simulink model "Amp_baseline1"  (R2020a)
settings: Solver=ode45  StartTime=0.0  StopTime=60  RelTol=1e-3
model workspace (MAT data in the model file):
  cfg_native : object (value not decoded)
  en_add_channels = 1
  host_ip = 2130706433
  host_port = 50223
  local_ip = 2130706433
  local_port = 50224
  num_en_channels = 32
  num_samples = 1
  sample_rate = 250
  serial_number = 'NB-2015.10.93'
undefined symbols (not defined in the file or in its folder): A1, A138674, A30722, currentCFG_Amp_baseline_UB, D1, fdesignblkfcn, gcbh, I1, J138674, N30722, UB
libraries: gtecHighspeedLib x14, dspfdesign x3, dsparch4 x2, dspstat3 x1, TobiiEyeTrackerLib x1, gUSBamplib x1
settings Model: ModifiedByFormat=g.tec  Creator=g.tec medical engineering  LastModifiedBy=g.tec
settings DataIOCC: LimitDataPoints=on  SaveFormat=Array  ReturnWorkspaceOutputs=off
settings OptimizationCC: BlockReduction=off  BooleanDataType=off  LifeSpan=inf
settings DebuggingCC: SaveWithParameterizedLinksMsg=none  UnderspecifiedInitializationDetection=Classic  MergeDetectMultiDrivingBlocksExec=none  SignalResolutionControl=TryResolveAllWithWarning  FrameProcessingCompatibilityMsg=none  SFUnexpectedBacktrackingDiag=warning  SFNoUnconditionalDefaultTransitionDiag=warning  SFExecutionAtInitializationDiag=none  ArithmeticOperatorsInVariantConditions=warning
settings HardwareCC: ProdBitPerPointer=32  ProdBitPerSizeT=32  ProdBitPerPtrDiffT=32  ProdLargestAtomicFloat=None  ProdIntDivRoundTo=Undefined  ProdEndianess=Unspecified  ProdWordSize=32  ProdHWDeviceType=32-bit Generic  TargetUnknown=on
settings ModelReferenceCC: PropagateSignalLabelsOutOfModel=off
settings SFSimCC: SimUseLocalCustomCode=off  CustomCodeUndefinedFunction=UseInterfaceOnly
settings RTWCC: RTWUseLocalCustomCode=off
settings CodeAppCC: StateflowObjectComments=on
settings GRTTargetCC: TargetLangStandard=C89/C90 (ANSI)
settings ConfigComp: CovMetricSettings=dw  CovHtmlReporting=on  CovSaveCumulativeToWorkspaceVar=on  CovSaveSingleToWorkspaceVar=on  CovExternalEMLEnable=off

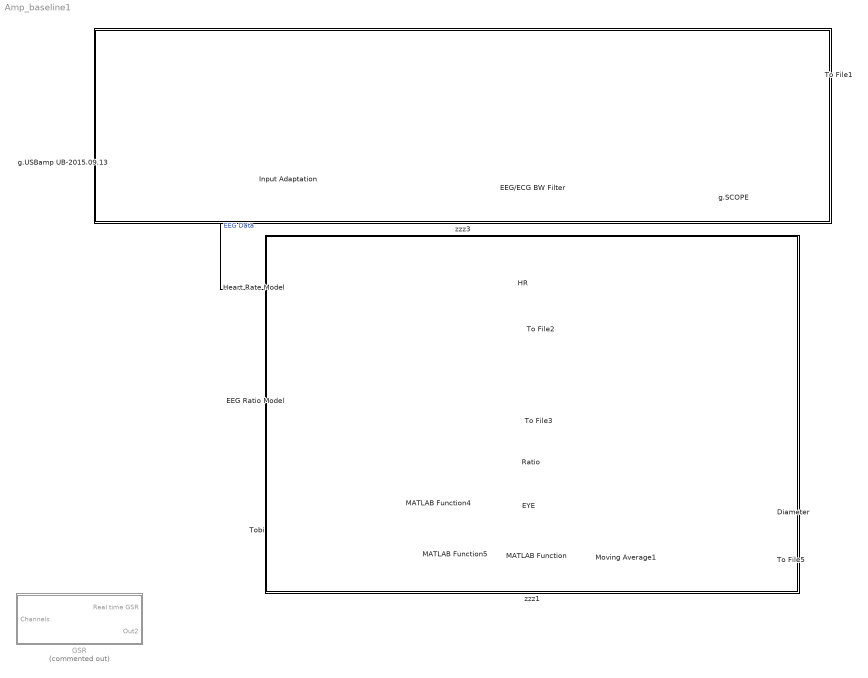
== system Amp_baseline1 ==
  Diameter : Display
  EEG Ratio Model : Subsystem
  EEG/ECG BW Filter : gtecHighspeedLib/EEG//ECG BW Filter  Order=6  LowerFreq=0.1  UpperFreq=30  SampFreq=512
      settings: SourceProductName=g.HIsys Library
  EYE : Display
  GSR : Subsystem  Commented=on
  HR : Display
  Heart Rate Model : ModelReference  ModelNameDialog=Heart_Rate_Model_Test  SimulationMode=Normal  ModelReferenceVersion=2.18.00
  Input Adaptation : Subsystem
  MATLAB Function : MATLAB Function  TreatAsAtomicUnit=on
  MATLAB Function4 : MATLAB Function  TreatAsAtomicUnit=on
  MATLAB Function5 : MATLAB Function  TreatAsAtomicUnit=on
  Moving Average1 : dspstat3/Moving Average  Method=Sliding window  ForgettingFactorPort=off  SpecifyWindowLength=on  WindowLength=512  ForgettingFactor=0.9  SimulateUsing=Code generation
  Ratio : Display
  To File1 : ToFile  Filename=Baseline.mat  MatrixName=Baselinedata
  To File2 : ToFile  Filename=Heartrate_Test.mat  MatrixName=heartRatedata
  To File3 : ToFile  Filename=Ratio.mat  MatrixName=Ratio
  To File5 : ToFile  Filename=Eye_Diameter.mat  MatrixName=Eye_Diameter
  Tobi : Subsystem
  g.SCOPE : gtecHighspeedLib/g.SCOPE
      settings: SourceProductName=g.HIsys Library
  g.USBamp UB-2015.09.13 : gUSBamplib/g.USBamp  cfg=currentCFG_Amp_baseline_UB-2015.09.13.cfg  snr=UB-2015.09.13
      settings: SourceProductName=g.USBamp
  zzz1 : Subsystem  TreatAsAtomicUnit=on
      settings: OpenFcn=% no-op
      mask Display: disp('')
  zzz3 : Subsystem  TreatAsAtomicUnit=on
      settings: OpenFcn=% no-op
      mask Display: disp('')
  wires:
  g.USBamp UB-2015.09.13/1 -> Input Adaptation/1(In), Heart Rate Model/1, EEG Ratio Model/1(Channels)  "EEG Data"
  Input Adaptation/1(Out) -> To File1/1, EEG/ECG BW Filter/1
  EEG/ECG BW Filter/1 -> g.SCOPE/1
  MATLAB Function/1(y) -> Moving Average1/1
  Moving Average1/1 -> To File5/1, Diameter/1
  MATLAB Function4/1(y) -> EYE/1, MATLAB Function/1(u)
  MATLAB Function5/1(y) -> MATLAB Function/2(Pupil_diameter_Left_Excel)
  EEG Ratio Model/2(Ratio Excel) -> Ratio/1, To File3/1
  Heart Rate Model/2 -> To File2/1
  Heart Rate Model/1 -> HR/1
  Tobi/2(Pupil diameter Right Excel) -> MATLAB Function4/1(Pupil_diameter_Right)
  Tobi/3(Pupil diameter Left Excel) -> MATLAB Function5/1(Pupil_diameter_Left)

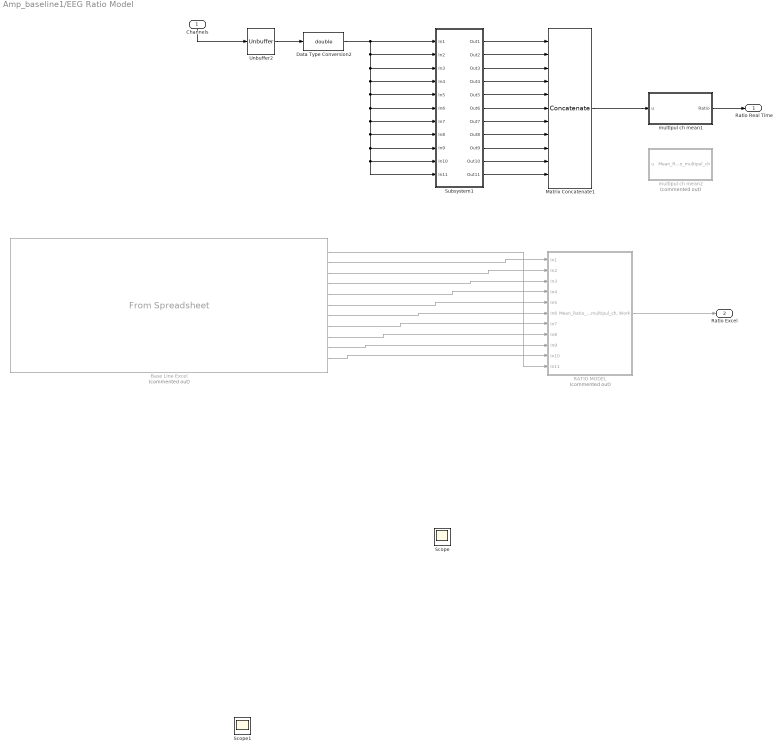
== system Amp_baseline1/EEG Ratio Model ==
  Channels : Inport
  Base Line Excel : FromSpreadsheet  Commented=on  FileName=C:\Users\LAB-OREN3\Downloads\1\Baseline Data of A2_535986.xlsx  SheetName=גיליון1  Range=A1:A30722,D1:N30722  SampleTime=0.001953125
  Data Type Conversion2 : DataTypeConversion  OutDataTypeStr=double
  Matrix Concatenate1 : Concatenate  NumInputs=11  Mode=Multidimensional array  ConcatenateDimension=2
  RATIO MODEL : Subsystem  Commented=on
  Scope : Scope
  Scope1 : Scope
  Subsystem1 : Subsystem
  Unbuffer2 : Unbuffer
  multipul ch mean1 : MATLAB Function  TreatAsAtomicUnit=on
  multipul ch mean2 : MATLAB Function  Commented=on  TreatAsAtomicUnit=on
  Ratio Real Time : Outport
  Ratio Excel : Outport  Port=2
  wires:
  Channels/1 -> Unbuffer2/1
  Matrix Concatenate1/1 -> multipul ch mean1/1(u)
  Subsystem1/4(Out4) -> Matrix Concatenate1/4
  Subsystem1/11(Out11) -> Matrix Concatenate1/11
  Subsystem1/8(Out8) -> Matrix Concatenate1/8
  Subsystem1/7(Out7) -> Matrix Concatenate1/7
  Subsystem1/6(Out6) -> Matrix Concatenate1/6
  Subsystem1/10(Out10) -> Matrix Concatenate1/10
  Subsystem1/3(Out3) -> Matrix Concatenate1/3
  Subsystem1/9(Out9) -> Matrix Concatenate1/9
  Unbuffer2/1 -> Data Type Conversion2/1
  Subsystem1/2(Out2) -> Matrix Concatenate1/2
  Subsystem1/5(Out5) -> Matrix Concatenate1/5
  Data Type Conversion2/1 -> Subsystem1/1(In1), Subsystem1/3(In3), Subsystem1/4(In4), Subsystem1/11(In11), Subsystem1/10(In10), Subsystem1/9(In9), Subsystem1/8(In8), Subsystem1/7(In7), Subsystem1/6(In6), Subsystem1/5(In5), Subsystem1/2(In2)
  Subsystem1/1(Out1) -> Matrix Concatenate1/1
  Base Line Excel/1 -> RATIO MODEL/11(In11)
  Base Line Excel/2 -> RATIO MODEL/1(In1)
  Base Line Excel/3 -> RATIO MODEL/2(In2)
  Base Line Excel/4 -> RATIO MODEL/3(In3)
  Base Line Excel/5 -> RATIO MODEL/4(In4)
  Base Line Excel/6 -> RATIO MODEL/5(In5)
  Base Line Excel/7 -> RATIO MODEL/6(In6)
  Base Line Excel/8 -> RATIO MODEL/7(In7)
  Base Line Excel/9 -> RATIO MODEL/8(In8)
  Base Line Excel/10 -> RATIO MODEL/9(In9)
  Base Line Excel/11 -> RATIO MODEL/10(In10)
  RATIO MODEL/1("Mean_Ratio_multipul_ch, Work") -> Ratio Excel/1
  multipul ch mean1/1(Ratio) -> Ratio Real Time/1

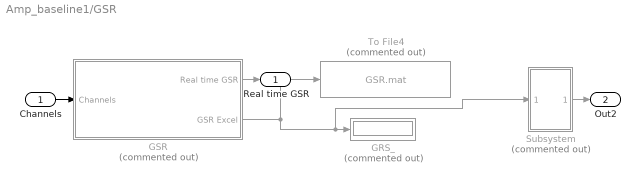
== system Amp_baseline1/GSR ==
  Channels : Inport
  GRS_ : Display  Commented=on
  GSR : Subsystem  Commented=on
  Subsystem : Subsystem  Commented=on
  To File4 : ToFile  Commented=on  Filename=GSR.mat  MatrixName=GSR
  Real time GSR : Outport
  Out2 : Outport  Port=2
  wires:
  GSR/2(GSR Excel) -> Subsystem/1(In1), GRS_/1, To File4/1
  Channels/1 -> GSR/1(Channels)
  GSR/1(Real time GSR) -> Real time GSR/1
  Subsystem/1(Out1) -> Out2/1

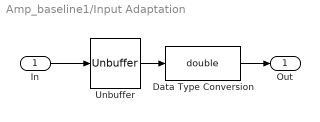
== system Amp_baseline1/Input Adaptation ==
  In : Inport
  Data Type Conversion : DataTypeConversion  OutDataTypeStr=double
  Unbuffer : Unbuffer
  Out : Outport
  wires:
  In/1 -> Unbuffer/1
  Unbuffer/1 -> Data Type Conversion/1
  Data Type Conversion/1 -> Out/1

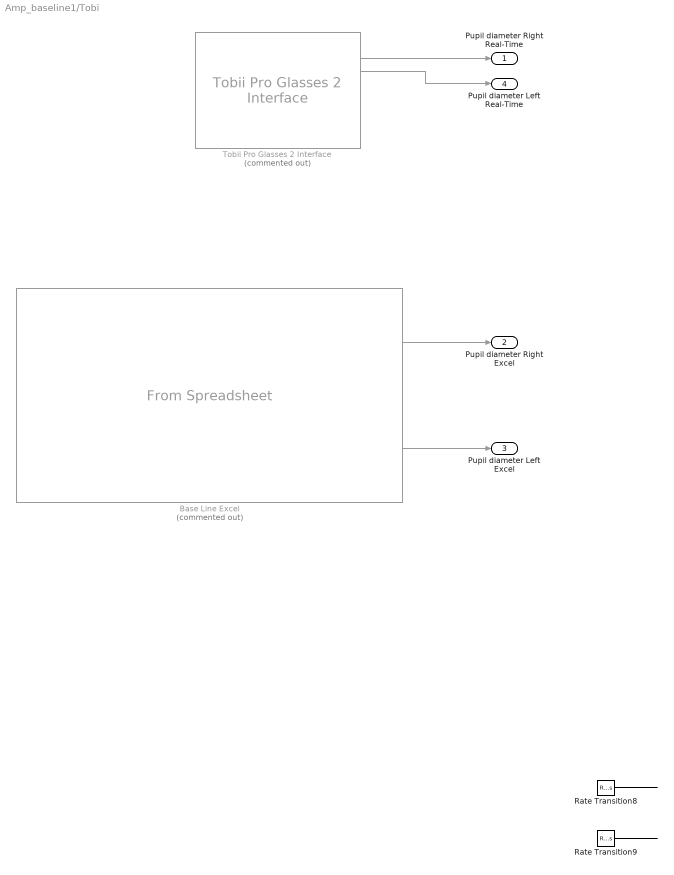
== system Amp_baseline1/Tobi ==
  Base Line Excel : FromSpreadsheet  Commented=on  FileName=C:\Users\LAB-OREN3\Desktop\CognataData\Participants_DATA\Test\4\Tobii Data of A1_546053_TRAINING at (12;02;18).xlsx  SheetName=גיליון1  Range=A1:A138674,I1:J138674  SampleTime=0.001953125
  Rate Transition8 : RateTransition  Deterministic=off  OutPortSampleTimeOpt=Inherit
  Rate Transition9 : RateTransition  Deterministic=off  OutPortSampleTimeOpt=Inherit
  Tobii Pro Glasses 2 Interface : TobiiEyeTrackerLib/Tobii Pro Glasses 2 Interface  Commented=on  Key=0  pc_right=off  pc_left=off  pd_right=off  pd_left=off  gd_right=off  gd_left=off  gp=on  gp3=off  gy=off  ac=off
      settings: SourceProductName=g.EYEtracking Interface (Tobii Pro Glasses 2)
  Pupil diameter Right Real-Time : Outport
  Pupil diameter Right Excel : Outport  Port=2
  Pupil diameter Left Excel : Outport  Port=3
  Pupil diameter Left Real-Time : Outport  Port=4
  wires:
  Rate Transition9/1 -> ?
  Rate Transition8/1 -> ?
  Tobii Pro Glasses 2 Interface/3 -> Pupil diameter Right Real-Time/1
  Base Line Excel/1 -> Pupil diameter Right Excel/1
  Base Line Excel/2 -> Pupil diameter Left Excel/1
  Tobii Pro Glasses 2 Interface/4 -> Pupil diameter Left Real-Time/1

== system Amp_baseline1/zzz1 ==

== system Amp_baseline1/zzz3 ==

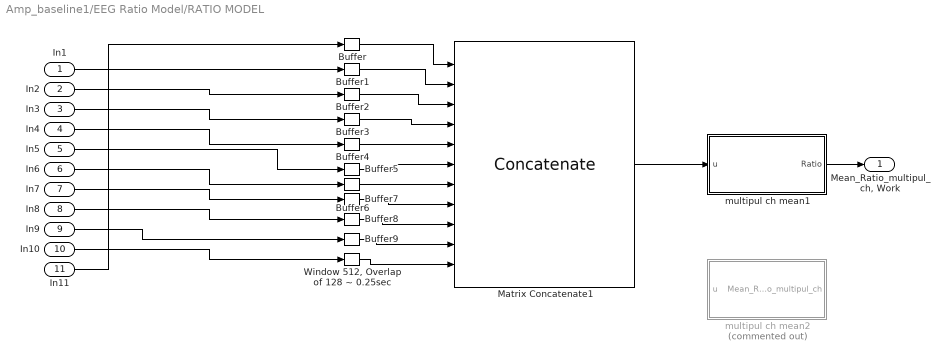
== system Amp_baseline1/EEG Ratio Model/RATIO MODEL ==
  In1 : Inport
  In2 : Inport  Port=2
  In3 : Inport  Port=3
  In4 : Inport  Port=4
  In5 : Inport  Port=5
  In6 : Inport  Port=6
  In7 : Inport  Port=7
  In8 : Inport  Port=8
  In9 : Inport  Port=9
  In10 : Inport  Port=10
  In11 : Inport  Port=11
  Buffer{,1..9} (10 alike) : Buffer  N=1536  V=1280  OutputFrames=off
  Matrix Concatenate1 : Concatenate  NumInputs=11  Mode=Multidimensional array  ConcatenateDimension=2
  "Window 512, Overlap of 128 ~ 0.25sec" : Buffer  N=1536  V=1280  OutputFrames=off
  multipul ch mean1 : MATLAB Function  TreatAsAtomicUnit=on
  multipul ch mean2 : MATLAB Function  Commented=on  TreatAsAtomicUnit=on
  "Mean_Ratio_multipul_ch, Work" : Outport
  wires:
  Buffer6/1 -> Matrix Concatenate1/7
  "Window 512, Overlap of 128 ~ 0.25sec"/1 -> Matrix Concatenate1/11
  Buffer3/1 -> Matrix Concatenate1/4
  Buffer2/1 -> Matrix Concatenate1/3
  Buffer4/1 -> Matrix Concatenate1/5
  Buffer5/1 -> Matrix Concatenate1/6
  Buffer/1 -> Matrix Concatenate1/1
  Buffer8/1 -> Matrix Concatenate1/9
  Buffer9/1 -> Matrix Concatenate1/10
  Buffer7/1 -> Matrix Concatenate1/8
  In7/1 -> Buffer7/1
  In10/1 -> "Window 512, Overlap of 128 ~ 0.25sec"/1
  Buffer1/1 -> Matrix Concatenate1/2
  In5/1 -> Buffer5/1
  In2/1 -> Buffer2/1
  In4/1 -> Buffer4/1
  In9/1 -> Buffer9/1
  In8/1 -> Buffer8/1
  In1/1 -> Buffer1/1
  In3/1 -> Buffer3/1
  In6/1 -> Buffer6/1
  In11/1 -> Buffer/1
  Matrix Concatenate1/1 -> multipul ch mean1/1(u)
  multipul ch mean1/1(Ratio) -> "Mean_Ratio_multipul_ch, Work"/1

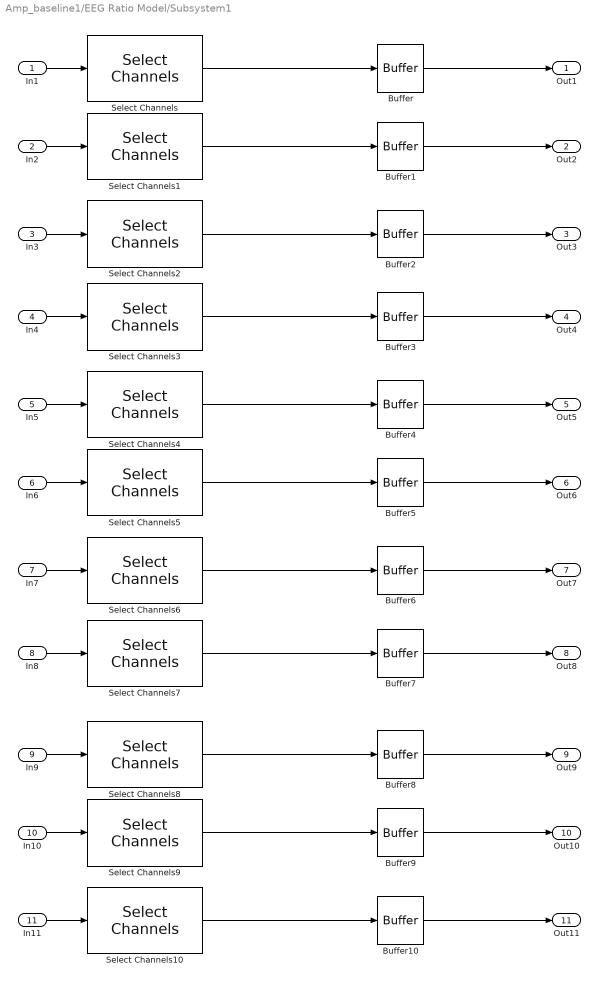
== system Amp_baseline1/EEG Ratio Model/Subsystem1 ==
  In1 : Inport
  In2 : Inport  Port=2
  In3 : Inport  Port=3
  In4 : Inport  Port=4
  In5 : Inport  Port=5
  In6 : Inport  Port=6
  In7 : Inport  Port=7
  In8 : Inport  Port=8
  In9 : Inport  Port=9
  In10 : Inport  Port=10
  In11 : Inport  Port=11
  Buffer{,1..10} (11 alike) : Buffer  N=512  V=384  OutputFrames=off
  Select Channels : gtecHighspeedLib/Select Channels  selectedchannels=[3]  totalchannels=14
      settings: SourceProductName=g.HIsys Library
  Select Channels1 : gtecHighspeedLib/Select Channels  selectedchannels=[4]  totalchannels=14
      settings: SourceProductName=g.HIsys Library
  Select Channels10 : gtecHighspeedLib/Select Channels  selectedchannels=[13]  totalchannels=14
      settings: SourceProductName=g.HIsys Library
  Select Channels2 : gtecHighspeedLib/Select Channels  selectedchannels=[5]  totalchannels=14
      settings: SourceProductName=g.HIsys Library
  Select Channels3 : gtecHighspeedLib/Select Channels  selectedchannels=[6]  totalchannels=14
      settings: SourceProductName=g.HIsys Library
  Select Channels4 : gtecHighspeedLib/Select Channels  selectedchannels=[7]  totalchannels=14
      settings: SourceProductName=g.HIsys Library
  Select Channels5 : gtecHighspeedLib/Select Channels  selectedchannels=[8]  totalchannels=14
      settings: SourceProductName=g.HIsys Library
  Select Channels6 : gtecHighspeedLib/Select Channels  selectedchannels=[9]  totalchannels=14
      settings: SourceProductName=g.HIsys Library
  Select Channels7 : gtecHighspeedLib/Select Channels  selectedchannels=[10]  totalchannels=14
      settings: SourceProductName=g.HIsys Library
  Select Channels8 : gtecHighspeedLib/Select Channels  selectedchannels=[11]  totalchannels=14
      settings: SourceProductName=g.HIsys Library
  Select Channels9 : gtecHighspeedLib/Select Channels  selectedchannels=[12]  totalchannels=14
      settings: SourceProductName=g.HIsys Library
  Out1 : Outport
  Out2 : Outport  Port=2
  Out3 : Outport  Port=3
  Out4 : Outport  Port=4
  Out5 : Outport  Port=5
  Out6 : Outport  Port=6
  Out7 : Outport  Port=7
  Out8 : Outport  Port=8
  Out9 : Outport  Port=9
  Out10 : Outport  Port=10
  Out11 : Outport  Port=11
  wires:
  In1/1 -> Select Channels/1
  Select Channels/1 -> Buffer/1
  In2/1 -> Select Channels1/1
  Select Channels1/1 -> Buffer1/1
  Buffer/1 -> Out1/1
  Buffer1/1 -> Out2/1
  Select Channels3/1 -> Buffer3/1
  Buffer3/1 -> Out4/1
  Select Channels2/1 -> Buffer2/1
  In4/1 -> Select Channels3/1
  In3/1 -> Select Channels2/1
  Buffer2/1 -> Out3/1
  Buffer6/1 -> Out7/1
  In8/1 -> Select Channels7/1
  In6/1 -> Select Channels5/1
  Select Channels7/1 -> Buffer7/1
  In5/1 -> Select Channels4/1
  Buffer4/1 -> Out5/1
  In7/1 -> Select Channels6/1
  Select Channels6/1 -> Buffer6/1
  Select Channels5/1 -> Buffer5/1
  Select Channels4/1 -> Buffer4/1
  Buffer7/1 -> Out8/1
  Buffer5/1 -> Out6/1
  In10/1 -> Select Channels9/1
  In9/1 -> Select Channels8/1
  Buffer10/1 -> Out11/1
  Buffer8/1 -> Out9/1
  Buffer9/1 -> Out10/1
  Select Channels9/1 -> Buffer9/1
  Select Channels10/1 -> Buffer10/1
  In11/1 -> Select Channels10/1
  Select Channels8/1 -> Buffer8/1

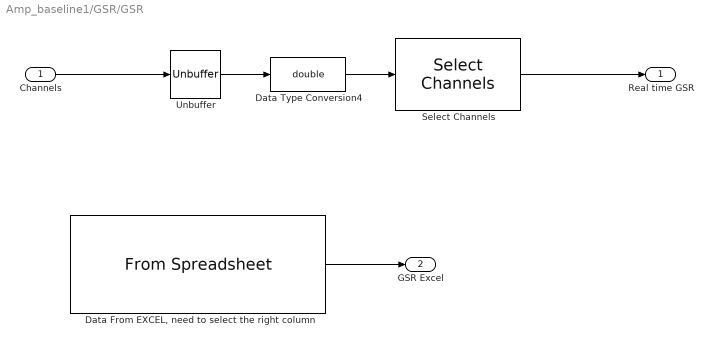
== system Amp_baseline1/GSR/GSR ==
  Channels : Inport
  "Data From EXCEL, need to select the right column " : FromSpreadsheet  FileName=C:\Users\LAB-OREN3\Desktop\CognataData\Participants_DATA\Nadav_Test\Physiological\Baseline Data of Nadav_Test\Baseline Data of Nadav_Test.xlsx  SheetName=גיליון1  Range=A1:B30722  SampleTime=0.001953125
  Data Type Conversion4 : DataTypeConversion  OutDataTypeStr=double
  Select Channels : gtecHighspeedLib/Select Channels  selectedchannels=[1]  totalchannels=14
      settings: SourceProductName=g.HIsys Library
  Unbuffer : Unbuffer
  Real time GSR : Outport
  GSR Excel : Outport  Port=2
  wires:
  Channels/1 -> Unbuffer/1
  Unbuffer/1 -> Data Type Conversion4/1
  Data Type Conversion4/1 -> Select Channels/1
  Select Channels/1 -> Real time GSR/1
  "Data From EXCEL, need to select the right column "/1 -> GSR Excel/1

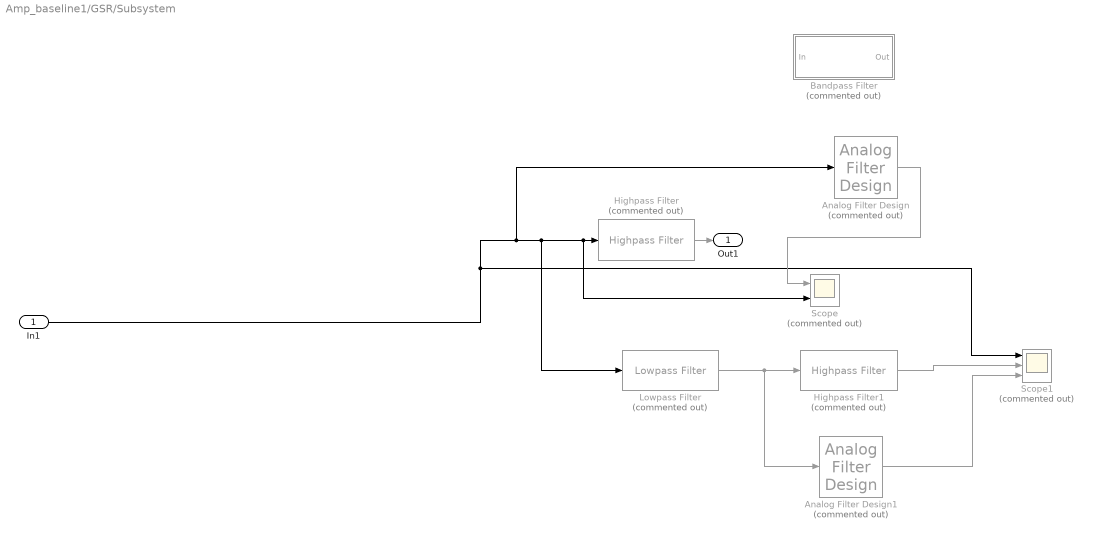
== system Amp_baseline1/GSR/Subsystem ==
  In1 : Inport
  Analog Filter Design : dsparch4/Analog Filter Design  Commented=on  method=Butterworth  filttype=Highpass  N=8  Wlo=0.05  Whi=80  Rp=2  Rs=40
  Analog Filter Design1 : dsparch4/Analog Filter Design  Commented=on  method=Butterworth  filttype=Highpass  N=50  Wlo=0.0001953125  Whi=80  Rp=2  Rs=40
  Bandpass Filter : Subsystem  Commented=on  DialogController=fdesignblkfcn  InitFcn=fdesignblkfcn(gcbh, {'InitFcn'});  mask(Bandpass Filter){}
      mask help: Design a bandpass filter
      settings: CopyFcn=fdesignblkfcn(gcbh, {'CopyFcn'});
      mask Help: helpview(mapfilelocation('dsp'), 'dspbandpassfilter');
      mask Display: disp('Bandpass');
  Highpass Filter : dspfdesign/Highpass Filter  Commented=on  FilterType=FIR  DesignForMinimumOrder=off  FilterOrder=50  StopbandFrequency=0.05  PassbandFrequency=0.05  StopbandAttenuation=80  PassbandRipple=0.1  InheritSampleRate=off  SampleRate=512  SimulateUsing=Interpreted execution  roundingMode=Floor  coeffsDataTypeStr=fixdt(1,16)
  Highpass Filter1 : dspfdesign/Highpass Filter  Commented=on  FilterType=FIR  DesignForMinimumOrder=off  FilterOrder=50  StopbandFrequency=8e3  PassbandFrequency=1  StopbandAttenuation=80  PassbandRipple=0.1  InheritSampleRate=on  SampleRate=512  SimulateUsing=Interpreted execution  roundingMode=Floor  coeffsDataTypeStr=fixdt(1,16)
  Lowpass Filter : dspfdesign/Lowpass Filter  Commented=on  FilterType=FIR  DesignForMinimumOrder=off  FilterOrder=50  PassbandFrequency=5  StopbandFrequency=12e3  PassbandRipple=0.1  StopbandAttenuation=80  InheritSampleRate=on  SampleRate=512  SimulateUsing=Interpreted execution  roundingMode=Floor  coeffsDataTypeStr=fixdt(1,16)
  Scope : Scope  Commented=on  NumInputPorts=2
  Scope1 : Scope  Commented=on  NumInputPorts=3
  Out1 : Outport
  wires:
  Lowpass Filter/1 -> Analog Filter Design1/1, Highpass Filter1/1
  In1/1 -> Analog Filter Design/1, Lowpass Filter/1, Scope/2, Highpass Filter/1, Scope1/1
  Highpass Filter/1 -> Out1/1
  Analog Filter Design1/1 -> Scope1/3
  Analog Filter Design/1 -> Scope/1
  Highpass Filter1/1 -> Scope1/2

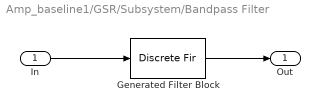
== system Amp_baseline1/GSR/Subsystem/Bandpass Filter ==
  In : Inport
  Generated Filter Block : DiscreteFir  Tag=BlockMethodSubSystem  Coefficients=[-0.0008992291487744296 0.0016414518747943749 0.0031352071842225397 -0.0040707550828814922 -0.0063731852227904111 0.0074874286806090491 0.0098354319566295711 -0.010189316513446216 -0.011302794465874122 0.0096929185841818435 0.0079428653987464216 -0.0031368247881221642 0.0028299878877943137 -0.011508674243001471 -0.022080136219461581 0.034245325424507672 0.048356661648905473 -0.062355369169884239 -0.077503478162593897 0.090687768153125653 0.10353171105844157 -0.11297860084229834 -0.12035866024978455 0.12379360801539134 0.12379360801539134 -0.12035866024978455 -0.11297860084229834 0.10353171105844157 0.090687768153125653 -0.077503478162593897 -0.062355369169884239 0.048356661648905473 0.034245325424507672 -0.022080136219461581 -0.011508674243001471 0.0028299878877943137 -0.0031368247881221642 0.0079428653987464216 0.0096929185841818435 -0.011302794465874122 -0.010189316513446216 0.0098354319566295711 0.0074874286806090491 -0.0063731852227904111 -0.0040707550828814922 0.0031352071842225397 0.0016414518747943749 -0.0008992291487744296]  InputProcessing=Columns as channels (frame based)
  Out : Outport  VectorParamsAs1DForOutWhenUnconnected=off
  wires:
  In/1 -> Generated Filter Block/1
  Generated Filter Block/1 -> Out/1

== matlab function Amp_baseline1/EEG Ratio Model/RATIO MODEL/multipul ch mean1 ==
  data: u input; Ratio output
function Ratio = EEG_Stress_Ratio(u)

Ratio= eeg_stress_ratio(u);


end

== matlab function Amp_baseline1/MATLAB Function ==
  data: u input; y output; Pupil_diameter_Left_Excel input
function y = fcn(u, Pupil_diameter_Left_Excel)
 
    
y = (u+Pupil_diameter_Left_Excel)/2;

== matlab function Amp_baseline1/EEG Ratio Model/RATIO MODEL/multipul ch mean2 ==
  data: u input; Mean_Ratio_multipul_ch output
function Mean_Ratio_multipul_ch = EEG_Stress_Ratio(u)

   coder.extrinsic('pwelch');
   coder.extrinsic('table2array');
   sampling_rate = 512;
   psd = zeros(513,1);
   frequencies = zeros(513,1);

   
   % On a 512 sampling rate we should have 129 freqwencies: to Obtain the Welch PSD estimate dividing the signal into segments 132 samples in length. The signal segments are multiplied by a Hamming window 132 samples in length. The number of overlapped samples is not specified, so it is set to 132/2 = 66. The DFT length is 256 points, yielding a frequency resolution of  rad/sample. Because the signal is real-valued, the PSD estimate is one-sided and there are 256/2+1 = 129 points. Plot the PSD as a function of normalized frequency.
   % 
%    number_of_frquencies = (size(u, 1)/4)+1;
%    disp(number_of_frquencies);
%    psd = zeros(number_of_frquencies,1);
%    frequencies = zeros(number_of_frquencies,1);
  
   %initialize an array to store the stress scores for each channel
   stress_scores = zeros(size(u, 2), 1);
   
   
       for i = 1:size(u, 2)
            
           %extract for current channel
           channel_data = u(:, i);
%            disp(channel_data);
            
          % Calculate the power spectral density (PSD) of the EEG data
           [psd, frequencies] = pwelch(channel_data, [], [], [], sampling_rate);
%             disp("psd test");
%             disp(psd);


           % Calculate the relative power in the alpha frequency band (8-12 Hz)
           alpha_power = sum(psd(frequencies >= 8 & frequencies <= 12)) / sum(psd);
%            disp("alpha_power");
%            disp(alpha_power);  
           
           % Calculate the relative power in the beta frequency band (12-30 Hz)
           beta_power = sum(psd(frequencies >= 12 & frequencies <= 30)) / sum(psd);
%            disp("beta_power");
%            disp(beta_power);  
           % Calculate the alpha/beta ratio for the current channel
%            alpha_beta_ratio = beta_power / alpha_power ;
             alpha_beta_ratio = log(beta_power/alpha_power) ;


            stress_scores(i) = alpha_beta_ratio;
            
            
       end
  
 
    Mean_Ratio_multipul_ch = mean(stress_scores);
end

== matlab function Amp_baseline1/EEG Ratio Model/multipul ch mean2 ==
  data: u input; Mean_Ratio_multipul_ch output
function Mean_Ratio_multipul_ch = EEG_Stress_Ratio(u)

   coder.extrinsic('pwelch');
   coder.extrinsic('table2array');
   sampling_rate = 512;
   % On a 512 sampling rate we should have 129 freqwencies: to Obtain the Welch PSD estimate dividing the signal into segments 132 samples in length. The signal segments are multiplied by a Hamming window 132 samples in length. The number of overlapped samples is not specified, so it is set to 132/2 = 66. The DFT length is 256 points, yielding a frequency resolution of  rad/sample. Because the signal is real-valued, the PSD estimate is one-sided and there are 256/2+1 = 129 points. Plot the PSD as a function of normalized frequency.
   % 
   number_of_frquencies = (size(u, 1)/4)+1;
   psd = zeros(number_of_frquencies,1);
   frequencies = zeros(number_of_frquencies,1);
  
   %initialize an array to store the stress scores for each channel
   stress_scores = zeros(size(u, 2), 1);
   
   
       for i = 1:size(u, 2)
            
           %extract for current channel
           channel_data = u(:, i);
            
           % Calculate the power spectral density (PSD) of the EEG data
           [psd, frequencies] = pwelch(channel_data, [], [], [], sampling_rate);


           % Calculate the relative power in the alpha frequency band (8-12 Hz)
           alpha_power = sum(psd(frequencies >= 8 & frequencies <= 12)) / sum(psd);

           % Calculate the relative power in the beta frequency band (12-30 Hz)
           beta_power = sum(psd(frequencies >= 12 & frequencies <= 30)) / sum(psd);

           % Calculate the alpha/beta ratio for the current channel
%            alpha_beta_ratio = beta_power / alpha_power ;
             alpha_beta_ratio = log(beta_power) - log(alpha_power) ;


            stress_scores(i) = alpha_beta_ratio;
            
       end
  
 
    Mean_Ratio_multipul_ch = mean(stress_scores);
end

== matlab function Amp_baseline1/EEG Ratio Model/multipul ch mean1 ==
  data: u input; Ratio output
function Ratio = EEG_Stress_Ratio(u)

Ratio= eeg_stress_ratio(u);


end

== matlab function Amp_baseline1/MATLAB Function4 ==
  data: Pupil_diameter_Right input; y output
function y = fcn(Pupil_diameter_Right)
    
  if Pupil_diameter_Right < 2.5 
      y = 2.5;
  elseif Pupil_diameter_Right > 8.0
      y = 8.0;
  else
      y = Pupil_diameter_Right;
  end
end

== matlab function Amp_baseline1/MATLAB Function5 ==
  data: Pupil_diameter_Left input; y output
function y = fcn(Pupil_diameter_Left)
    
  if Pupil_diameter_Left < 2.5 
      y = 2.5;
  elseif Pupil_diameter_Left > 8.0
      y = 8.0;
  else
      y = Pupil_diameter_Left;
  end
end
